simulink model "webcam_storage_test3"  (Simulink 7.3)
settings: Solver=FixedStepDiscrete  StartTime=0.0  StopTime=inf  MaxStep=0.2  RelTol=1e-3
settings Model: Creator=gclayton  LastModifiedBy=wildcat
settings DebuggingCC: InheritedTsInSrcMsg=none
settings RTWCC: SystemTargetFile=rlnx.tlc  GenCodeOnly=on  TemplateMakefile=rlnx_ubuntu.tmf  Description=Linux Real-Time Target  ProcessScript=rlnx_make_rtw_hook
settings RTWCC: CustomInclude=|
  | /usr/local/include/opencv/
  | /usr/local/include/
settings CodeAppCC: GenerateComments=off  SimulinkBlockComments=off
settings STFCustomTargetCC: ModelReferenceCompliant=off  MatFileLogging=on  SystemTargetFile=rlnx.tlc
settings GRTTargetCC: ModelReferenceCompliant=off  ParMdlRefBuildCompliant=off  CompOptLevelCompliant=off
settings CustomProperty: DataType=string  Value=-lm -ldl /usr/local/lib/libopencv_highgui.so.2.4 /usr/local/lib/libopencv_core.so.2.4 /usr/local/lib/libopencv_imgproc.so.2.4
settings EnumStrPairs: String=PC

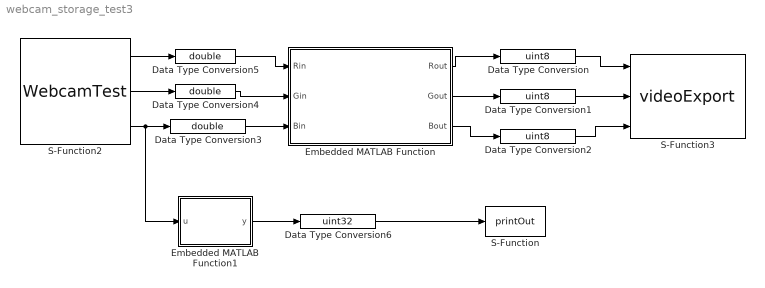
== system webcam_storage_test3 ==
  Data Type Conversion : DataTypeConversion  OutDataTypeMode=uint8  OutDataType=fixdt(1, 16)  OutScaling=2^0  OutDataTypeStr=uint8
  Data Type Conversion1 : DataTypeConversion  OutDataTypeMode=uint8  OutDataType=fixdt(1, 16)  OutScaling=2^0  OutDataTypeStr=uint8
  Data Type Conversion2 : DataTypeConversion  OutDataTypeMode=uint8  OutDataType=fixdt(1, 16)  OutScaling=2^0  OutDataTypeStr=uint8
  Data Type Conversion3 : DataTypeConversion  OutDataTypeMode=double  OutDataType=fixdt(1, 16)  OutScaling=2^0  OutDataTypeStr=double
  Data Type Conversion4 : DataTypeConversion  OutDataTypeMode=double  OutDataType=fixdt(1, 16)  OutScaling=2^0  OutDataTypeStr=double
  Data Type Conversion5 : DataTypeConversion  OutDataTypeMode=double  OutDataType=fixdt(1, 16)  OutScaling=2^0  OutDataTypeStr=double
  Data Type Conversion6 : DataTypeConversion  OutDataTypeMode=uint32  OutDataType=fixdt(1, 16)  OutScaling=2^0  OutDataTypeStr=uint32
  Embedded MATLAB Function : Stateflow chart
  Embedded MATLAB Function1 : Stateflow chart  TreatAsAtomicUnit=on
  S-Function : S-Function  FunctionName=printOut  EnableBusSupport=off
  S-Function2 : S-Function  FunctionName=WebcamTest  EnableBusSupport=off
  S-Function3 : S-Function  FunctionName=videoExport  EnableBusSupport=off
  wires:
  S-Function2/1 -> Data Type Conversion5/1
  S-Function2/2 -> Data Type Conversion4/1
  S-Function2/3 -> Data Type Conversion3/1, Embedded MATLAB Function1/1(u)
  Embedded MATLAB Function/1(Rout) -> Data Type Conversion/1
  Data Type Conversion/1 -> S-Function3/1
  Embedded MATLAB Function/2(Gout) -> Data Type Conversion1/1
  Data Type Conversion1/1 -> S-Function3/2
  Embedded MATLAB Function/3(Bout) -> Data Type Conversion2/1
  Data Type Conversion2/1 -> S-Function3/3
  Data Type Conversion3/1 -> Embedded MATLAB Function/3(Bin)
  Data Type Conversion4/1 -> Embedded MATLAB Function/2(Gin)
  Data Type Conversion5/1 -> Embedded MATLAB Function/1(Rin)
  Data Type Conversion6/1 -> S-Function/1
  Embedded MATLAB Function1/1(y) -> Data Type Conversion6/1

== matlab function Embedded MATLAB Function1 ==
  data: u input double; y output double
function y = fcn(u)

y = u(100,100);

== matlab function Embedded MATLAB Function ==
  data: Rin input double; Rout output double; Gin input double; Bin input double; Gout output double; Bout output double
function [Rout, Gout, Bout] = videoExport_format(Rin,Gin,Bin)
% Format information from block properly in order to export

Rout = zeros(1,307200);
Bout = zeros(1,307200);
Gout = zeros(1,307200);

for i = 1:640
    for j = 1:480
        Rout(j+480*(i-1)) = Rin(j,i);
        Gout(j+480*(i-1)) = Gin(j,i);
        Bout(j+480*(i-1)) = Bin(j,i);
    end
    
end
